simulink model "autopilota_v_15_last"  (R2020b)
settings: Solver=ode4  StartTime=0.0  StopTime=300  FixedStep=0.02  RelTol=1e-3
values from neighbouring files (symbols this model uses):
  attuatore_Amax = 20*(pi/180)    (= 0.349065850399)    [v2021_10_27_avvioSITL.m]    (also in v2021_10_27_calcoloAerodinamica.m)
  attuatore_Amin = -20*(pi/180)    (= -0.349065850399)    [v2021_10_27_avvioSITL.m]
  attuatore_Emax = 25*(pi/180)    (= 0.436332312999)    [v2021_10_27_avvioSITL.m]    (also in v2021_10_27_calcoloAerodinamica.m)
  attuatore_Emin = -25*(pi/180)    (= -0.436332312999)    [v2021_10_27_avvioSITL.m]
  attuatore_Rmax = 25*(pi/180)    (= 0.436332312999)    [v2021_10_27_avvioSITL.m]    (also in v2021_10_27_calcoloAerodinamica.m)
  attuatore_Rmin = -25*(pi/180)    (= -0.436332312999)    [v2021_10_27_avvioSITL.m]
  attuatore_Tmax = 0.99    [v2021_10_27_avvioSITL.m]
  attuatore_Tmin = 0    [v2021_10_27_avvioSITL.m]
  bias = [baccxINI,baccyINI,bacczINI,bpINI,bqINI,brINI]    [v2021_10_27_avvioSITL.m]
  final_h = 35    [v2021_10_27_avvioSITL.m]
  interventoA_05 = 20*0.8    (= 16)    [v2021_10_27_avvioSITL.m]
  interventoA_1 = 10    [v2021_10_27_avvioSITL.m]
  interventoE_05 = 25*0.8    (= 20)    [v2021_10_27_avvioSITL.m]
  interventoE_1 = 10    [v2021_10_27_avvioSITL.m]
  interventoT = 1*0.6    (= 0.6)    [v2021_10_27_avvioSITL.m]
  inv_A = 1    [v2021_10_27_avvioSITL.m]
  inv_comp_h = 1    [v2021_10_27_avvioSITL.m]
  inv_E = 1    [v2021_10_27_avvioSITL.m]
  inv_R = 1    [v2021_10_27_avvioSITL.m]
  inv_T = 1    [v2021_10_27_avvioSITL.m]
  K_AW_B_AP_quota = 1000    [v2021_10_27_avvioSITL.m]
  K_AW_B_becc = -250    [v2021_10_27_avvioSITL.m]
  K_AW_B_imb = 0    [v2021_10_27_avvioSITL.m]
  K_AW_B_roll = 500    [v2021_10_27_avvioSITL.m]
  K_imb_inv = -0.001306    [v2021_10_27_avvioSITL.m]
  Kd_AP_rotta = 0.995    [v2021_10_27_avvioSITL.m]
  Kd_h_app = 0.085    [v2021_10_27_avvioSITL.m]
  Kd_h_flare = 0.01    [v2021_10_27_avvioSITL.m]
  Ki_AP_quota_select = 0.01936    [v2021_10_27_avvioSITL.m]
  Ki_AP_rotta = 0.002    [v2021_10_27_avvioSITL.m]
  Ki_AP_vel = 0.025175    [v2021_10_27_avvioSITL.m]
  Ki_becch = -0.1963    [v2021_10_27_avvioSITL.m]
  Ki_h_app = 0.055    [v2021_10_27_avvioSITL.m]
  Ki_h_cruise = 0.008    [v2021_10_27_avvioSITL.m]
  Ki_h_flare = 0.07    [v2021_10_27_avvioSITL.m]
  Ki_roll = 0.004528    [v2021_10_27_avvioSITL.m]
  Kp_AP_quota_hold_h = 0.5503    [v2021_10_27_avvioSITL.m]
  Kp_AP_quota_hold_l = 0.5503    [v2021_10_27_avvioSITL.m]
  Kp_AP_quota_select = 0.02647    [v2021_10_27_avvioSITL.m]
  Kp_AP_rotta = 0.520    (= 0.52)    [v2021_10_27_avvioSITL.m]
  Kp_AP_vel = 0.132175    [v2021_10_27_avvioSITL.m]
  Kp_becch = -0.30    (= -0.3)    [v2021_10_27_avvioSITL.m]
  Kp_comp_h = 0.035    [v2021_10_27_avvioSITL.m]
  Kp_h_app_max = 0.086    [v2021_10_27_avvioSITL.m]
  Kp_h_app_min = 0.01    [v2021_10_27_avvioSITL.m]
  Kp_h_cruise = 0.04    [v2021_10_27_avvioSITL.m]
  Kp_h_flare = 0.1    [v2021_10_27_avvioSITL.m]
  Kp_imb = 0.0019415    [v2021_10_27_avvioSITL.m]
  Kp_p = 0.006913    [v2021_10_27_avvioSITL.m]
  Kp_q = -0.025    [v2021_10_27_avvioSITL.m]
  Kp_roll = 0.0718    [v2021_10_27_avvioSITL.m]
  Kp_Rotta_ATO = 4    [v2021_10_27_avvioSITL.m]
  Kp_Rotta_psi = -0.01    [v2021_10_27_avvioSITL.m]
  Q1B = [    2e-15;     2e-15 ... (first row only)    [COV_F1B.m]
  R1B = [     2e-14;             2e-14 ... (first row only)    [COV_F1B.m]
  safe_phi = 55    [v2021_10_27_avvioSITL.m]
  safe_V = 40    [v2021_10_27_avvioSITL.m]
  Sensor_Offsets = [0,0,0]    [v2021_10_27_avvioSITL.m]
  T_cal = 0.4    [v2021_10_27_avvioSITL.m]
  theta_rot = 10    [v2021_10_27_avvioSITL.m]
  time_alarm_SAFE = 300    [v2021_10_27_avvioSITL.m]
  tsamp = 0.02    [v2021_10_27_avvioSITL.m]
  update = [2,2,2]    [v2021_10_27_avvioSITL.m]
  V_max = 35    [v2021_10_27_avvioSITL.m]
  V_stall = 15    [v2021_10_27_avvioSITL.m]
  vd_ini = 0    [v2021_10_27_avvioSITL.m]
  vel_wp1_al = 25    [v2021_10_27_avvioSITL.m]
  vel_wp2_al = 20    [v2021_10_27_avvioSITL.m]
undefined symbols (not defined in the file or in its folder): DiscIntNeverNeededParam, Newton, Raphson, t_AP
libraries: simulink_extras x41, pid_lib x8, dspsigops x4, simulink x3, aerolibtransform2sys x2, aerolibtransform2 x2, cstblocks x1, aerosimlib x1
(part 9 of 11)

== matlab function autopilota_v_15_last/Subsystem1/Subsystem1/Subsystem2/WAYPOINTS3 ==
  data: lat input; long input; h input; psi input; WP_db_info input; e_h output; vel output; lat_comandato output; long_comandato output; distance output; QUOTA output; ROTTA output; WP_db_param input; GC_info input; counter input; counter_out output
% % % % function [e_h,vel,lat_comandato,long_comandato,distance,QUOTA,ROTTA,...
% % % %     counter_out] = waypoints_tracking(lat,long,h,psi,WP_db_info,...
% % % %     WP_db_param,GC_info,counter)
% % % % %#codegen
% % % % %WP_db_info=(nWP_tot , n_WP , frame , command , current , autocontinue)
% % % % %per Nav
% % % % %WP_db_param=(velocità, autocontinue, vuoto, vuoto, lat_comandato, ...
% % % % %long_comandato, h_comandato)
% % % % % 
% % % % persistent flag lat1 long1 
% % % % 
% % % % if isempty (flag)
% % % %     flag = 0;
% % % % end
% % % % if isempty (lat1)
% % % %     lat1 = 0;
% % % % end
% % % % if isempty (long1)
% % % %     long1=0;
% % % % end
% % % % 
% % % % % autocontinue = WP_db_param(counter,4);      
% % % % %se vale 1 si procede al waypoint successivo, 
% % % % %se vale 0 loitera sul waypoint
% % % % 
% % % % autocontinue = 1;
% % % % %se arrivo all'ultimo WP, loiter 
% % % % if counter == size(WP_db_param,1) && autocontinue > 0    
% % % %     autocontinue = 0;     
% % % % end
% % % % % if autocontinue >=1
% % % % %     autocontinue = 1;
% % % % % end
% % % % 
% % % % %se ricevo dei WP, comincio dal WP con il current
% % % % %altrimenti ricomincio dal WP1!!!
% % % % if GC_info==3
% % % %     counter=1;
% % % %     lat1=lat;
% % % %     long1=long;
% % % %     for indice=1:size(WP_db_param,1)
% % % %         if WP_db_info(indice,5)==1
% % % %             counter=indice;
% % % %         end
% % % %     end
% % % % end
% % % % 
% % % % %Definizione posizione waypoints
% % % % lat_comandato = WP_db_param(counter,5);
% % % % long_comandato = WP_db_param(counter,6);
% % % % h_comandato = WP_db_param(counter,7);
% % % % Rearth=6378137; %m
% % % % % e_lat = lat_comandato - lat;        %errore in gradi
% % % % % e_long = long_comandato - long;     %errore in gradi 
% % % % e_h = h_comandato - h;
% % % % 
% % % % a = (sin(((lat_comandato-lat)*pi/180)/2))^2+cos(lat*pi/180)*...
% % % %     cos(lat_comandato*pi/180)*(sin(((long_comandato-long)*pi/180)/2))^2;
% % % % c = 2*atan2(sqrt(a),sqrt(1-a));
% % % % distance = Rearth*c;               %distanza velivolo-WP
% % % % 
% % % % if counter > 1
% % % %     psi_ref = atan2(sin((WP_db_param(counter,6)-...
% % % %         WP_db_param(counter-1,6))*pi/180)*...
% % % %         cos(WP_db_param(counter,5)*pi/180),cos(WP_db_param(counter-1,5)...
% % % %         *pi/180)*sin(WP_db_param(counter,5)*pi/180)-...
% % % %         sin(WP_db_param(counter-1,5)*pi/180)*cos(WP_db_param(counter,5)...
% % % %         *pi/180)*cos((WP_db_param(counter,6)-WP_db_param(counter-1,6))...
% % % %         *pi/180))*180/pi;     %psi di riferimento
% % % % %    distWP = sqrt((6378137*(lat_comandato-WP_db_param(counter-1,5))...
% % % % %    *pi/180)^2 + (6378137*(long_comandato-WP_db_param(counter-1,6))...
% % % % %    *pi/180)^2);                          %distanza tra due WP successivi
% % % %     a_pre = (sin(((lat-WP_db_param(counter-1,5))*pi/180)/2))^2+...
% % % %         cos(WP_db_param(counter-1,5)*pi/180)*cos(lat*pi/180)*...
% % % %         (sin(((long-WP_db_param(counter-1,6))*pi/180)/2))^2;
% % % %     c_pre = 2*atan2(sqrt(a_pre),sqrt(1-a_pre));
% % % %     dist = Rearth*c_pre;                  %distanza velivolo-WP precedente
% % % % else
% % % %     psi_ref = atan2(sin((long_comandato-long1)*pi/180)*...
% % % %         cos(lat_comandato*pi/180),cos(lat1*pi/180)*...
% % % %         sin(lat_comandato*pi/180)-sin(lat1*pi/180)*...
% % % %         cos(lat_comandato*pi/180)*cos((long_comandato-long1)...
% % % %         *pi/180))*180/pi;
% % % % %    distWP = 6378137;
% % % %     dist = 0;
% % % % end
% % % % 
% % % % if psi_ref < 0
% % % %     psi_ref = 360 - abs(psi_ref);
% % % % end
% % % %       
% % % % 
% % % % %Definizione angolo tra WP successivi
% % % % if autocontinue == 1
% % % %     a_fut = (sin(((WP_db_param(counter+1,5)-WP_db_param(counter,5))...
% % % %         *pi/180)/2))^2+cos(WP_db_param(counter,5)*pi/180)...
% % % %         *cos(WP_db_param(counter+1,5)*pi/180)...
% % % %         *(sin(((WP_db_param(counter+1,6)-WP_db_param(counter,6))...
% % % %         *pi/180)/2))^2;
% % % %     c_fut = 2*atan2(sqrt(a_fut),sqrt(1-a_fut));
% % % %     dist_fut = 6378137*c_fut;
% % % %     psi_ref_fut = atan2(sin((WP_db_param(counter+1,6)-...
% % % %         WP_db_param(counter,6))*pi/180)*cos(WP_db_param(counter+1,5)...
% % % %         *pi/180),cos(WP_db_param(counter,5)*pi/180)*...
% % % %         sin(WP_db_param(counter+1,5)*pi/180)-sin(WP_db_param(counter,5)...
% % % %         *pi/180)*cos(WP_db_param(counter+1,5)*pi/180)*...
% % % %         cos((WP_db_param(counter+1,6)-WP_db_param(counter,6))...
% % % %         *pi/180))*180/pi;      %distanza WP-WP+1
% % % %     if psi_ref_fut < 0
% % % %         psi_ref_fut = 360 - abs(psi_ref_fut);
% % % %     end
% % % %     if counter > 1
% % % %         angoloWP = abs(psi_ref_fut - psi_ref);
% % % %     else 
% % % %         angoloWP = abs(psi_ref_fut - (atan2(sin((long_comandato-long1)...
% % % %             *pi/180)*cos(lat_comandato*pi/180),cos(lat1*pi/180)*...
% % % %             sin(lat_comandato*pi/180)-sin(lat1*pi/180)*...
% % % %             cos(lat_comandato*pi/180)*cos((long_comandato-long1)...
% % % %             *pi/180))*180/pi));
% % % %     end
% % % % else
% % % %     dist_fut = 0;
% % % %     angoloWP = 0;
% % % % end
% % % % 
% % % % 
% % % % 
% % % % if counter < 2
% % % %     angoloWP_pre = 0;
% % % % elseif counter == 2
% % % %     angoloWP_pre = abs(psi_ref - atan2(sin((WP_db_param(counter-1,6)...
% % % %         -long1)*pi/180)*cos(WP_db_param(counter-1,5)*pi/180),...
% % % %         cos(lat1*pi/180)*sin(WP_db_param(counter-1,5)*pi/180)...
% % % %         -sin(lat1*pi/180)*cos(WP_db_param(counter-1,5)*pi/180)...
% % % %         *cos((WP_db_param(counter-1,6)-long1)*pi/180))*180/pi);
% % % % else
% % % %     psi_ref_pre = atan2(sin((WP_db_param(counter-1,6)-...
% % % %         WP_db_param(counter-2,6))*pi/180)*cos(WP_db_param(counter-1,5)...
% % % %         *pi/180),cos(WP_db_param(counter-2,5)*pi/180)*...
% % % %         sin(WP_db_param(counter-1,5)*pi/180)-...
% % % %         sin(WP_db_param(counter-2,5)*pi/180)*...
% % % %         cos(WP_db_param(counter-1,5)*pi/180)*...
% % % %         cos((WP_db_param(counter-1,6)-WP_db_param(counter-2,6))...
% % % %         *pi/180))*180/pi;
% % % % if psi_ref_pre < 0
% % % %     psi_ref_pre = 360 - abs(psi_ref_pre);
% % % % end
% % % %     angoloWP_pre = abs(psi_ref - psi_ref_pre);
% % % % end
% % % %     
% % % % 
% % % % if angoloWP <= 10
% % % %     error = 40;                            %Definizione raggio di errore 
% % % %     tolleranza_distWP_fut = 100;           %Definizione distanza minima... 
% % % % elseif angoloWP > 10 && angoloWP <= 50     %accettabile tra WP successivi
% % % %     error = 60;
% % % %     tolleranza_distWP_fut = 250;
% % % % elseif angoloWP > 50 && angoloWP <= 90     
% % % %     error = 80;
% % % %     tolleranza_distWP_fut = 300;
% % % % elseif angoloWP > 90 && angoloWP <= 120     
% % % %     error = 120;
% % % %     tolleranza_distWP_fut = 350;
% % % % else     
% % % %     error = 150;
% % % %     tolleranza_distWP_fut = 400;
% % % % end
% % % % 
% % % % %Protezione WP troppo vicini
% % % % % for i=1 : size(WP_db_param,1)-1
% % % % %     a_fut(i) = (sin(((WP_db_param(i+1,5)-WP_db_param(i,5))*pi/180)/2))^2+cos(WP_db_param(i,5)*pi/180)*cos(WP_db_param(i+1,5)*pi/180)*(sin(((WP_db_param(i+1,6)-WP_db_param(i,6))*pi/180)/2))^2;
% % % % %     c_fut(i) = 2*atan2(sqrt(a_fut(i)),sqrt(1-a_fut(i)));
% % % % %     dist_fut(i) = 6378137*c_fut(i);
% % % % %     if dist_fut(i) <= tolleranza_distWP_fut
% % % % %         WP_db_param(i+1,:) = [];
% % % % %     end
% % % % % end
% % % % 
% % % % nWP=size(WP_db_param,1);
% % % % 
% % % % if angoloWP_pre <= 10
% % % % %     tolleranza_distWP = 100;                          
% % % %     soglia_dist = 50;%Distanza dal WP precedente per correzione traiettoria
% % % % elseif angoloWP_pre > 10 && angoloWP_pre <= 50 
% % % % %     tolleranza_distWP = 250;
% % % %     soglia_dist = 200;
% % % % elseif angoloWP_pre > 50 && angoloWP_pre <= 90 
% % % % %     tolleranza_distWP = 300;
% % % %     soglia_dist = 300;
% % % % elseif angoloWP_pre > 90 && angoloWP_pre <= 120 
% % % % %     tolleranza_distWP = 350;
% % % %     soglia_dist = 350;
% % % % else
% % % % %     tolleranza_distWP = 400;
% % % %     soglia_dist = 400;
% % % % end
% % % % 
% % % % k=1.3;    %fattore moltiplicativo correzione rotta
% % % % 
% % % % %Definizione rotta
% % % % 
% % % % if autocontinue == 1
% % % %     
% % % %     psi_comandato = atan2(sin((long_comandato - long)*pi/180)*...
% % % %         cos(lat_comandato*pi/180),cos(lat*pi/180)*...
% % % %         sin(lat_comandato*pi/180)-sin(lat*pi/180)*...
% % % %         cos(lat_comandato*pi/180)*cos((long_comandato - long)...
% % % %         *pi/180))*180/pi;     %rotta da seguire
% % % %     vel = WP_db_param(counter,3);    %??     %inserisci velocità desiderata 
% % % %     psi_comandato_fut = atan2(sin((WP_db_param(counter+1,6)-long)...
% % % %         *pi/180)*cos(WP_db_param(counter+1,5)*pi/180),cos(lat*pi/180)...
% % % %         *sin(WP_db_param(counter+1,5)*pi/180)-sin(lat*pi/180)...
% % % %         *cos(WP_db_param(counter+1,5)*pi/180)...
% % % %         *cos((WP_db_param(counter+1,6)-long)*pi/180))*180/pi;
% % % %     if vel < 15
% % % %         vel = 25;
% % % %     end
% % % %     
% % % %     if vel <= 20%Definizione raggio di errore in base alla velocità di volo
% % % %         error = error*1;
% % % %     elseif (vel <= 25 && vel > 20)
% % % %         error = error*1.2;
% % % %     elseif (vel <= 30 && vel > 25)
% % % %         error = error*1.3;
% % % %     else 
% % % %         error = error*1.4;
% % % %     end
% % % %     
% % % % %         psi_comandato = atan2(sin((long_comandato - long)*pi/180)...
% % % % %             *cos(lat_comandato*pi/180),cos(lat*pi/180)...
% % % % %             *sin(lat_comandato*pi/180)-sin(lat*pi/180)...
% % % % %             *cos(lat_comandato*pi/180)*cos((long_comandato - long)...
% % % % %             *pi/180))*180/pi;    %già dichiarata
% % % % %         if dist < soglia_dist && distance > error
% % % % %             psi_comandato = atan2(sin((long_comandato - long)*pi/180)...
% % % % %                 *cos(lat_comandato*pi/180),cos(lat*pi/180)...
% % % % %                 *sin(lat_comandato*pi/180)-sin(lat*pi/180)...
% % % % %                 *cos(lat_comandato*pi/180)*cos((long_comandato - long)...
% % % % %                 *pi/180))*180/pi;
% % % %          if dist > soglia_dist && distance > error
% % % %             psi_comandato = atan2(sin((long_comandato - long)*pi/180)...
% % % %                 *cos(lat_comandato*pi/180),cos(lat*pi/180)...
% % % %                 *sin(lat_comandato*pi/180)-sin(lat*pi/180)...
% % % %                 *cos(lat_comandato*pi/180)*cos((long_comandato - long)...
% % % %                 *pi/180))*180/pi;
% % % %             err = abs ( psi_comandato - psi_ref );%errore inseguimento rotta
% % % %             if (psi_ref <= 90 && psi_ref >= 0)    %primo quadrante
% % % %                 if psi_comandato > psi_ref
% % % %                     psi_comandato = psi_comandato + k*err;
% % % %                 elseif psi_comandato < psi_ref
% % % %                     psi_comandato = psi_comandato - k*err;
% % % %                 else
% % % %                     psi_comandato = psi_comandato;
% % % %                 end                   
% % % %             elseif (psi_ref <= 180 && psi_ref > 90)   %secondo quadrante
% % % %                 if psi_ref*psi_comandato > 0
% % % %                     if psi_comandato > psi_ref || ( psi_comandato < -90 ...
% % % %                             && psi_comandato > -180)
% % % %                         psi_comandato = psi_comandato + k*err;
% % % %                     elseif psi_comandato < psi_ref
% % % %                         psi_comandato = psi_comandato - k*err;
% % % %                     else
% % % %                         psi_comandato = psi_comandato;
% % % %                     end                      
% % % %                 else
% % % %                     err = abs ( 360 - abs(psi_comandato) - psi_ref); 
% % % %                     if psi_comandato > psi_ref || ( psi_comandato < -90 ...
% % % %                             && psi_comandato > -180)
% % % %                         psi_comandato = psi_comandato + k*err;
% % % %                     elseif psi_comandato < psi_ref
% % % %                         psi_comandato = psi_comandato - k*err;
% % % %                     else
% % % %                         psi_comandato = psi_comandato;
% % % %                     end                     
% % % %                 end
% % % %             elseif(psi_ref < -90 && psi_ref >= -180)       %terzo quadrante
% % % %                 if psi_ref*psi_comandato > 0
% % % %                     if psi_comandato > psi_ref
% % % %                         psi_comandato = psi_comandato + k*err;
% % % %                     elseif psi_comandato < psi_ref  || (psi_comandato <...
% % % %                             180 && psi_comandato > 90)
% % % %                         psi_comandato = psi_comandato - k*err;
% % % %                     else
% % % %                         psi_comandato = psi_comandato;
% % % %                     end  
% % % %                 else
% % % %                     err = abs ( 360 -(psi_comandato) - abs(psi_ref)); 
% % % %                     if psi_comandato > psi_ref
% % % %                         psi_comandato = psi_comandato + k*err;
% % % %                     elseif psi_comandato < psi_ref || (psi_comandato <...
% % % %                             180 && psi_comandato > 90)
% % % %                         psi_comandato = psi_comandato - k*err;
% % % %                     else
% % % %                         psi_comandato = psi_comandato;
% % % %                     end                     
% % % %                 end
% % % %             elseif(psi_ref < 0 && psi_ref >= -90)       %quarto quadrante
% % % %                 if psi_comandato > psi_ref
% % % %                     psi_comandato = psi_comandato + k*err;
% % % %                 elseif psi_comandato < psi_ref
% % % %                     psi_comandato = psi_comandato - k*err;
% % % %                 else
% % % %                     psi_comandato = psi_comandato;
% % % %                 end
% % % %             end
% % % %             
% % % %         elseif distance < error
% % % %             if dist_fut > tolleranza_distWP_fut
% % % %                 psi_comandato = psi_comandato_fut;
% % % %                 counter = counter + 1;
% % % %             else
% % % %                 if counter < nWP-1
% % % %                     counter = counter + 2;
% % % %                 else
% % % %                     vel=22;
% % % %                     h_comandato=h+0.4;
% % % %                     psi_comandato=psi+36.6;   
% % % %                     e_h=0;
% % % %                     flag=1;
% % % %                 end
% % % %             end
% % % %         end
% % % %             
% % % %     flag = 0;
% % % %     
% % % % else
% % % %     
% % % %     psi_comandato = atan2(sin((long_comandato - long)*pi/180)...
% % % %         *cos(lat_comandato*pi/180),cos(lat*pi/180)...
% % % %         *sin(lat_comandato*pi/180)-sin(lat*pi/180)...
% % % %         *cos(lat_comandato*pi/180)*cos((long_comandato - long)...
% % % %         *pi/180))*180/pi;
% % % %     vel = WP_db_param(counter,3);        %inserisci velocità desiderata
% % % %     error = 40;
% % % %     if vel < 15
% % % %         vel = 25;
% % % %     end
% % % %     
% % % %         if dist < soglia_dist && flag == 0
% % % %                   psi_comandato = atan2(sin((long_comandato - long)...
% % % %                       *pi/180)*cos(lat_comandato*pi/180),...
% % % %                       cos(lat*pi/180)*sin(lat_comandato*pi/180)...
% % % %                       -sin(lat*pi/180)*cos(lat_comandato*pi/180)...
% % % %                       *cos((long_comandato - long)*pi/180))*180/pi;
% % % %         elseif dist > soglia_dist && distance > error && flag == 0
% % % %                 err = abs ( psi_comandato - psi_ref );        
% % % %                 if (psi_ref <= 90 && psi_ref >= 0)       %primo quadrante
% % % %                     if psi_comandato > psi_ref
% % % %                         psi_comandato = psi_comandato + k*err;
% % % %                     elseif psi_comandato < psi_ref
% % % %                         psi_comandato = psi_comandato - k*err;
% % % %                     else
% % % %                         psi_comandato = psi_comandato;
% % % %                     end 
% % % %                 elseif (psi_ref <= 180 && psi_ref > 90)  %secondo quadrante
% % % %                     if psi_ref*psi_comandato > 0
% % % %                         if psi_comandato > psi_ref || ( psi_comandato <...
% % % %                                 -90 && psi_comandato > -180)
% % % %                             psi_comandato = psi_comandato + k*err;
% % % %                         elseif psi_comandato < psi_ref
% % % %                             psi_comandato = psi_comandato - k*err;
% % % %                         else
% % % %                             psi_comandato = psi_comandato;
% % % %                         end
% % % %                     else
% % % %                         err = abs ( 360 - abs(psi_comandato) - psi_ref); 
% % % %                         if psi_comandato > psi_ref || ( psi_comandato <...
% % % %                                 -90 && psi_comandato > -180)
% % % %                             psi_comandato = psi_comandato + k*err;
% % % %                         elseif psi_comandato < psi_ref
% % % %                             psi_comandato = psi_comandato - k*err;
% % % %                         else
% % % %                             psi_comandato = psi_comandato;
% % % %                         end                     
% % % %                     end
% % % %                 elseif(psi_ref < -90 && psi_ref >= -180)   %terzo quadrante
% % % %                     if psi_ref*psi_comandato > 0
% % % %                         if psi_comandato > psi_ref
% % % %                             psi_comandato = psi_comandato + k*err;
% % % %                         elseif psi_comandato < psi_ref  || ...
% % % %                                 (psi_comandato < 180 && psi_comandato > 90)
% % % %                             psi_comandato = psi_comandato - k*err;
% % % %                         else
% % % %                             psi_comandato = psi_comandato;
% % % %                         end 
% % % %                     else
% % % %                         err = abs ( 360 -(psi_comandato) - abs(psi_ref)); 
% % % %                         if psi_comandato > psi_ref
% % % %                             psi_comandato = psi_comandato + k*err;
% % % %                         elseif psi_comandato < psi_ref || (psi_comandato...
% % % %                                 < 180 && psi_comandato > 90)
% % % %                             psi_comandato = psi_comandato - k*err;
% % % %                         else
% % % %                             psi_comandato = psi_comandato;
% % % %                         end                         
% % % %                     end
% % % %                 elseif(psi_ref < 0 && psi_ref >= -90) %quarto quadrante
% % % %                     if psi_comandato > psi_ref
% % % %                         psi_comandato = psi_comandato + k*err;
% % % %                     elseif psi_comandato < psi_ref
% % % %                         psi_comandato = psi_comandato - k*err;
% % % %                     else
% % % %                         psi_comandato = psi_comandato;
% % % %                     end
% % % %                 end
% % % %                 
% % % %         else            
% % % %                 vel=22;
% % % %                 h_comandato=h+0.4;
% % % %                 psi_comandato=psi+36.6;   
% % % %                 e_h=0;
% % % %                 flag=1;        %con flag=1 l'aereo rimane in loiter...             
% % % %         end                    %senza uscire dal ciclo
% % % %           
% % % % end
% % % % 
% % % % 
% % % % %se ho nWPtotali=0 (lat,long,alt==0), traiettoria circolare
% % % % if lat_comandato == 0 && long_comandato == 0 && h_comandato==0    
% % % %     h_comandato=h+0.3;
% % % %     psi_comandato=psi+36.6;   
% % % %     vel=22;
% % % %     e_h=0;   
% % % % end
% % % % 
% % % % %output  
% % % % QUOTA = h_comandato;
% % % % ROTTA = psi_comandato;
% % % % 
% % % % counter_out=counter;



function [e_h,vel,lat_comandato,long_comandato,distance,QUOTA,ROTTA,counter_out] = waypoints_tracking(lat,long,h,psi,WP_db_info,WP_db_param,GC_info,counter)
%#codegen
%WP_db_info=(nWP_tot n_WP frame command current autocontinue)
%per Nav
%WP_db_param=(velocità, autocontinue, vuoto, vuoto, lat_comandato, long_comandato, h_comandato)

persistent flag lat1 long1 

if isempty (flag)
    flag = 0;
end
if isempty (lat1)
    lat1 = 0;
end
if isempty (long1)
    long1=0;
end

% autocontinue = WP_db_param(counter,4);      %se vale 1 si procede al waypoint successivo, se vale 0 loitera sul waypoint

autocontinue = 1;
%se arrivo all'ultimo WP, loiter 
if counter == size(WP_db_param,1) && autocontinue > 0    
    autocontinue = 0;     
end
% if autocontinue >=1
%     autocontinue = 1;
% end

%se ricevo dei WP, comincio dal WP con il current
%altrimenti ricomincio dal WP1!!!
if GC_info==3
    counter=1;
    lat1=lat;
    long1=long;
    for indice=1:size(WP_db_param,1)
        if WP_db_info(indice,5)==1
            counter=indice;
        end
    end
end

%Definizione posizione waypoints
lat_comandato = WP_db_param(counter,5);
long_comandato = WP_db_param(counter,6);
h_comandato = WP_db_param(counter,7);

% e_lat = lat_comandato - lat;        %errore in gradi
% e_long = long_comandato - long;     %errore in gradi 
e_h = h_comandato - h;

a = (sin(((lat_comandato-lat)*pi/180)/2))^2+cos(lat*pi/180)*cos(lat_comandato*pi/180)*(sin(((long_comandato-long)*pi/180)/2))^2;
c = 2*atan2(sqrt(a),sqrt(1-a));
distance = 6378137*c;               %distanza velivolo-WP

if counter > 1
    psi_ref = atan2(sin((WP_db_param(counter,6)-WP_db_param(counter-1,6))*pi/180)*cos(WP_db_param(counter,5)*pi/180),cos(WP_db_param(counter-1,5)*pi/180)*sin(WP_db_param(counter,5)*pi/180)-sin(WP_db_param(counter-1,5)*pi/180)*cos(WP_db_param(counter,5)*pi/180)*cos((WP_db_param(counter,6)-WP_db_param(counter-1,6))*pi/180))*180/pi;     %psi di riferimento
%    distWP = sqrt((6378137*(lat_comandato-WP_db_param(counter-1,5))*pi/180)^2 + (6378137*(long_comandato-WP_db_param(counter-1,6))*pi/180)^2);                                          %distanza tra due WP successivi
    a_pre = (sin(((lat-WP_db_param(counter-1,5))*pi/180)/2))^2+cos(WP_db_param(counter-1,5)*pi/180)*cos(lat*pi/180)*(sin(((long-WP_db_param(counter-1,6))*pi/180)/2))^2;
    c_pre = 2*atan2(sqrt(a_pre),sqrt(1-a_pre));
    dist = 6378137*c_pre;                                                  %distanza velivolo-WP precedente
else
    psi_ref = atan2(sin((long_comandato-long1)*pi/180)*cos(lat_comandato*pi/180),cos(lat1*pi/180)*sin(lat_comandato*pi/180)-sin(lat1*pi/180)*cos(lat_comandato*pi/180)*cos((long_comandato-long1)*pi/180))*180/pi;
%    distWP = 6378137;
    dist = 0;
end

if psi_ref < 0
    psi_ref = 360 - abs(psi_ref);
end
      

%Definizione angolo tra WP successivi
if autocontinue == 1
    a_fut = (sin(((WP_db_param(counter+1,5)-WP_db_param(counter,5))*pi/180)/2))^2+cos(WP_db_param(counter,5)*pi/180)*cos(WP_db_param(counter+1,5)*pi/180)*(sin(((WP_db_param(counter+1,6)-WP_db_param(counter,6))*pi/180)/2))^2;
    c_fut = 2*atan2(sqrt(a_fut),sqrt(1-a_fut));
    dist_fut = 6378137*c_fut;
    psi_ref_fut = atan2(sin((WP_db_param(counter+1,6)-WP_db_param(counter,6))*pi/180)*cos(WP_db_param(counter+1,5)*pi/180),cos(WP_db_param(counter,5)*pi/180)*sin(WP_db_param(counter+1,5)*pi/180)-sin(WP_db_param(counter,5)*pi/180)*cos(WP_db_param(counter+1,5)*pi/180)*cos((WP_db_param(counter+1,6)-WP_db_param(counter,6))*pi/180))*180/pi;      %distanza WP-WP+1
    if psi_ref_fut < 0
        psi_ref_fut = 360 - abs(psi_ref_fut);
    end
    if counter > 1
        angoloWP = abs(psi_ref_fut - psi_ref);
    else 
        angoloWP = abs(psi_ref_fut - (atan2(sin((long_comandato-long1)*pi/180)*cos(lat_comandato*pi/180),cos(lat1*pi/180)*sin(lat_comandato*pi/180)-sin(lat1*pi/180)*cos(lat_comandato*pi/180)*cos((long_comandato-long1)*pi/180))*180/pi));
    end
else
    dist_fut = 0;
    angoloWP = 0;
end



if counter < 2
    angoloWP_pre = 0;
elseif counter == 2
    angoloWP_pre = abs(psi_ref - atan2(sin((WP_db_param(counter-1,6)-long1)*pi/180)*cos(WP_db_param(counter-1,5)*pi/180),cos(lat1*pi/180)*sin(WP_db_param(counter-1,5)*pi/180)-sin(lat1*pi/180)*cos(WP_db_param(counter-1,5)*pi/180)*cos((WP_db_param(counter-1,6)-long1)*pi/180))*180/pi);
else
    psi_ref_pre = atan2(sin((WP_db_param(counter-1,6)-WP_db_param(counter-2,6))*pi/180)*cos(WP_db_param(counter-1,5)*pi/180),cos(WP_db_param(counter-2,5)*pi/180)*sin(WP_db_param(counter-1,5)*pi/180)-sin(WP_db_param(counter-2,5)*pi/180)*cos(WP_db_param(counter-1,5)*pi/180)*cos((WP_db_param(counter-1,6)-WP_db_param(counter-2,6))*pi/180))*180/pi;
if psi_ref_pre < 0
    psi_ref_pre = 360 - abs(psi_ref_pre);
end
    angoloWP_pre = abs(psi_ref - psi_ref_pre);
end
    

if angoloWP <= 10
    error = 40;                                       %Definizione raggio di errore 
    tolleranza_distWP_fut = 100;                      %Definizione distanza minima accettabile tra WP successivi
elseif angoloWP > 10 && angoloWP <= 50 
    error = 60;
    tolleranza_distWP_fut = 250;
elseif angoloWP > 50 && angoloWP <= 90     
    error = 80;
    tolleranza_distWP_fut = 300;
elseif angoloWP > 90 && angoloWP <= 120     
    error = 120;
    tolleranza_distWP_fut = 350;
else     
    error = 150;
    tolleranza_distWP_fut = 400;
end

%Protezione WP troppo vicini
% for i=1 : size(WP_db_param,1)-1
%     a_fut(i) = (sin(((WP_db_param(i+1,5)-WP_db_param(i,5))*pi/180)/2))^2+cos(WP_db_param(i,5)*pi/180)*cos(WP_db_param(i+1,5)*pi/180)*(sin(((WP_db_param(i+1,6)-WP_db_param(i,6))*pi/180)/2))^2;
%     c_fut(i) = 2*atan2(sqrt(a_fut(i)),sqrt(1-a_fut(i)));
%     dist_fut(i) = 6378137*c_fut(i);
%     if dist_fut(i) <= tolleranza_distWP_fut
%         WP_db_param(i+1,:) = [];
%     end
% end

nWP=size(WP_db_param,1);

if angoloWP_pre <= 10
%     tolleranza_distWP = 100;                          
    soglia_dist = 50;                                   %Distanza dal WP precedente per correzione traiettoria
elseif angoloWP_pre > 10 && angoloWP_pre <= 50 
%     tolleranza_distWP = 250;
    soglia_dist = 200;
elseif angoloWP_pre > 50 && angoloWP_pre <= 90 
%     tolleranza_distWP = 300;
    soglia_dist = 300;
elseif angoloWP_pre > 90 && angoloWP_pre <= 120 
%     tolleranza_distWP = 350;
    soglia_dist = 350;
else
%     tolleranza_distWP = 400;
    soglia_dist = 400;
end

k=1.3;    %fattore moltiplicativo correzione rotta

%Definizione rotta

if autocontinue == 1
    
    psi_comandato = atan2(sin((long_comandato - long)*pi/180)*cos(lat_comandato*pi/180),cos(lat*pi/180)*sin(lat_comandato*pi/180)-sin(lat*pi/180)*cos(lat_comandato*pi/180)*cos((long_comandato - long)*pi/180))*180/pi;     %rotta da seguire
    vel = WP_db_param(counter,3);                   %inserisci velocità desiderata 
    psi_comandato_fut = atan2(sin((WP_db_param(counter+1,6)-long)*pi/180)*cos(WP_db_param(counter+1,5)*pi/180),cos(lat*pi/180)*sin(WP_db_param(counter+1,5)*pi/180)-sin(lat*pi/180)*cos(WP_db_param(counter+1,5)*pi/180)*cos((WP_db_param(counter+1,6)-long)*pi/180))*180/pi;
    if vel < 15
        vel = 25;
    end
    
    if vel <= 20                                    %Definizione raggio di errore in base alla velocità di volo
        error = error*1;
    elseif (vel <= 25 && vel > 20)
        error = error*1.2;
    elseif (vel <= 30 && vel > 25)
        error = error*1.3;
    else 
        error = error*1.4;
    end
    
        psi_comandato = atan2(sin((long_comandato - long)*pi/180)*cos(lat_comandato*pi/180),cos(lat*pi/180)*sin(lat_comandato*pi/180)-sin(lat*pi/180)*cos(lat_comandato*pi/180)*cos((long_comandato - long)*pi/180))*180/pi;    
        if dist < soglia_dist && distance > error
            psi_comandato = atan2(sin((long_comandato - long)*pi/180)*cos(lat_comandato*pi/180),cos(lat*pi/180)*sin(lat_comandato*pi/180)-sin(lat*pi/180)*cos(lat_comandato*pi/180)*cos((long_comandato - long)*pi/180))*180/pi;
        elseif dist > soglia_dist && distance > error
            psi_comandato = atan2(sin((long_comandato - long)*pi/180)*cos(lat_comandato*pi/180),cos(lat*pi/180)*sin(lat_comandato*pi/180)-sin(lat*pi/180)*cos(lat_comandato*pi/180)*cos((long_comandato - long)*pi/180))*180/pi;
            err = abs ( psi_comandato - psi_ref );             %errore inseguimento rotta
            if (psi_ref <= 90 && psi_ref >= 0)                 %primo quadrante
                if psi_comandato > psi_ref
                    psi_comandato = psi_comandato + k*err;
                elseif psi_comandato < psi_ref
                    psi_comandato = psi_comandato - k*err;
                else
                    psi_comandato = psi_comandato;
                end                   
            elseif (psi_ref <= 180 && psi_ref > 90)             %quarto quadrante
                if psi_ref*psi_comandato > 0
                    if psi_comandato > psi_ref || ( psi_comandato < -90 && psi_comandato > -180)
                        psi_comandato = psi_comandato + k*err;
                    elseif psi_comandato < psi_ref
                        psi_comandato = psi_comandato - k*err;
                    else
                        psi_comandato = psi_comandato;
                    end                      
                else
                    err = abs ( 360 - abs(psi_comandato) - psi_ref); 
                    if psi_comandato > psi_ref || ( psi_comandato < -90 && psi_comandato > -180)
                        psi_comandato = psi_comandato + k*err;
                    elseif psi_comandato < psi_ref
                        psi_comandato = psi_comandato - k*err;
                    else
                        psi_comandato = psi_comandato;
                    end                     
                end
            elseif(psi_ref < -90 && psi_ref >= -180)             %terzo quadrante
                if psi_ref*psi_comandato > 0
                    if psi_comandato > psi_ref
                        psi_comandato = psi_comandato + k*err;
                    elseif psi_comandato < psi_ref  || (psi_comandato < 180 && psi_comandato > 90)
                        psi_comandato = psi_comandato - k*err;
                    else
                        psi_comandato = psi_comandato;
                    end  
                else
                    err = abs ( 360 -(psi_comandato) - abs(psi_ref)); 
                    if psi_comandato > psi_ref
                        psi_comandato = psi_comandato + k*err;
                    elseif psi_comandato < psi_ref || (psi_comandato < 180 && psi_comandato > 90)
                        psi_comandato = psi_comandato - k*err;
                    else
                        psi_comandato = psi_comandato;
                    end                     
                end
            elseif(psi_ref < 0 && psi_ref >= -90)             %secondo quadrante
                if psi_comandato > psi_ref
                    psi_comandato = psi_comandato + k*err;
                elseif psi_comandato < psi_ref
                    psi_comandato = psi_comandato - k*err;
                else
                    psi_comandato = psi_comandato;
                end
            end
            
        elseif distance < error
            if dist_fut > tolleranza_distWP_fut
                psi_comandato = psi_comandato_fut;
                counter = counter + 1;
            else
                if counter < nWP-1
                    counter = counter + 2;
                else
                    vel=22;
                    h_comandato=h+0.4;
                    psi_comandato=psi+36.6;   
                    e_h=0;
                    flag=1;
                end
            end
        end
            
    flag = 0;
    
else
    
    psi_comandato = atan2(sin((long_comandato - long)*pi/180)*cos(lat_comandato*pi/180),cos(lat*pi/180)*sin(lat_comandato*pi/180)-sin(lat*pi/180)*cos(lat_comandato*pi/180)*cos((long_comandato - long)*pi/180))*180/pi;
    vel = WP_db_param(counter,3);                   %inserisci velocità desiderata
    error = 40;
    if vel < 15
        vel = 25;
    end
    
        if dist < soglia_dist && flag == 0
                  psi_comandato = atan2(sin((long_comandato - long)*pi/180)*cos(lat_comandato*pi/180),cos(lat*pi/180)*sin(lat_comandato*pi/180)-sin(lat*pi/180)*cos(lat_comandato*pi/180)*cos((long_comandato - long)*pi/180))*180/pi;
        elseif dist > soglia_dist && distance > error && flag == 0
                err = abs ( psi_comandato - psi_ref );        
                if (psi_ref <= 90 && psi_ref >= 0)                 %primo quadrante
                    if psi_comandato > psi_ref
                        psi_comandato = psi_comandato + k*err;
                    elseif psi_comandato < psi_ref
                        psi_comandato = psi_comandato - k*err;
                    else
                        psi_comandato = psi_comandato;
                    end 
                elseif (psi_ref <= 180 && psi_ref > 90)             %quarto quadrante
                    if psi_ref*psi_comandato > 0
                        if psi_comandato > psi_ref || ( psi_comandato < -90 && psi_comandato > -180)
                            psi_comandato = psi_comandato + k*err;
                        elseif psi_comandato < psi_ref
                            psi_comandato = psi_comandato - k*err;
                        else
                            psi_comandato = psi_comandato;
                        end
                    else
                        err = abs ( 360 - abs(psi_comandato) - psi_ref); 
                        if psi_comandato > psi_ref || ( psi_comandato < -90 && psi_comandato > -180)
                            psi_comandato = psi_comandato + k*err;
                        elseif psi_comandato < psi_ref
                            psi_comandato = psi_comandato - k*err;
                        else
                            psi_comandato = psi_comandato;
                        end                     
                    end
                elseif(psi_ref < -90 && psi_ref >= -180)             %terzo quadrante
                    if psi_ref*psi_comandato > 0
                        if psi_comandato > psi_ref
                            psi_comandato = psi_comandato + k*err;
                        elseif psi_comandato < psi_ref  || (psi_comandato < 180 && psi_comandato > 90)
                            psi_comandato = psi_comandato - k*err;
                        else
                            psi_comandato = psi_comandato;
                        end 
                    else
                        err = abs ( 360 -(psi_comandato) - abs(psi_ref)); 
                        if psi_comandato > psi_ref
                            psi_comandato = psi_comandato + k*err;
                        elseif psi_comandato < psi_ref || (psi_comandato < 180 && psi_comandato > 90)
                            psi_comandato = psi_comandato - k*err;
                        else
                            psi_comandato = psi_comandato;
                        end                         
                    end
                elseif(psi_ref < 0 && psi_ref >= -90)             %secondo quadrante
                    if psi_comandato > psi_ref
                        psi_comandato = psi_comandato + k*err;
                    elseif psi_comandato < psi_ref
                        psi_comandato = psi_comandato - k*err;
                    else
                        psi_comandato = psi_comandato;
                    end
                end
                
        else            
                vel=22;
                h_comandato=h+0.4;
                psi_comandato=psi+36.6;   
                e_h=0;
                flag=1;                       %con flag=1 l'aereo rimane in loiter senza uscire dal ciclo            
        end
          
end


%se ho nWPtotali=0 (lat,long,alt==0), traiettoria circolare
if lat_comandato == 0 && long_comandato == 0 && h_comandato==0    
    h_comandato=h+0.3;
    psi_comandato=psi+36.6;   
    vel=22;
    e_h=0;   
end

%output  
QUOTA = h_comandato;
ROTTA = psi_comandato;

counter_out=counter;





% function [e_h,vel,lat_comandato,long_comandato,distance,QUOTA,ROTTA,counter_out] = waypoints_tracking(lat,long,h,psi,WP_db_info,WP_db_param,GC_info,counter)
% %#codegen
% %WP_db_info=(nWP_tot n_WP frame command current autocontinue)
% %per Nav
% %WP_db_param=(velocità, autocontinue, vuoto, vuoto, lat_comandato, long_comandato, h_comandato)
% 
% persistent flag
% 
% if isempty(flag)
%     flag = 0;
% end
% 
% counter_out=counter;
% autocontinue = WP_db_param(counter,2);      %se vale 1 si procede al waypoint successivo, se vale 0 loitera sul waypoint
% 
% if autocontinue >=1
%     autocontinue = 1;
% end
% 
% %se ricevo dei WP, comincio dal WP con il current
% %altrimenti ricomincio dal WP1!!!
% if GC_info==3
%     counter=1;
%     for indice=1:size(WP_db_param,1)
%         if WP_db_info(indice,5)==1
%             counter=indice;
%         end
%     end
% end
% 
% %Definizione posizione waypoints
% lat_comandato = WP_db_param(counter,5);
% long_comandato = WP_db_param(counter,6);
% h_comandato = WP_db_param(counter,7);
% 
% e_lat = lat_comandato - lat;        %errore in gradi
% e_long = long_comandato - long;     %errore in gradi 
% e_h = h_comandato - h;
% 
% e_x=6378137*e_lat*pi/180;           %passo a errore di distanza   %prima si utilizzava per il raggio 6372800;
% e_y=6378137*e_long*pi/180;          %passo a errore di distanza
% distance=sqrt((e_x)^2 + (e_y)^2 + (e_h)^2);
% 
% if counter > 1   
%     psi_ref = atan2((6378137*(WP_db_param(counter,6)-WP_db_param(counter-1,6))*pi/180),(6378137*((WP_db_param(counter,5)-WP_db_param(counter-1,5))*pi/180))) *180/pi;
% else
%     psi_ref = atan2((e_y),(e_x)) *180/pi; 
% end
% 
% if counter > 1
%     dist = sqrt((6378137*(lat_comandato-WP_db_param(counter-1,5)))^2 + (6378137*(long_comandato-WP_db_param(counter-1,6)))^2);
% else
%     dist = 6378137;
% end
%          
% tolleranza_dist = 320;
% tolleranza_rotta_1 = 18;
% tolleranza_rotta_2 = 9;
% tolleranza_rotta_3 = 2;
% 
% %Definizione rotta
% 
% if autocontinue == 1
%     
%     psi_comandato = atan2((e_y),(e_x)) *180/pi; 
%     vel = WP_db_param(counter,1);         %inserisci velocità desiderata
%     
%     if vel <= 20                          %Definizione raggio di errore
%         error = 25;
%     elseif (vel <= 25 && vel > 20)
%         error = 30;
%     elseif (vel <= 30 && vel > 25)
%         error = 40;
%     else 
%         error = 45;
%     end
% 
%     if dist > tolleranza_dist 
%         
%         psi_comandato = atan2((e_y),(e_x)) *180/pi; 
%         
%         if distance >= error*3
%             
%             if (psi_ref <= 90 && psi_ref >= 0)                 %primo quadrante
%                 if abs(psi_comandato - psi_ref) > tolleranza_rotta_1
%                     if psi_comandato > psi_ref
%                         psi_comandato = psi_comandato + 35;
%                     else
%                         psi_comandato = psi_comandato - 35;
%                     end
%                 elseif abs(psi_comandato - psi_ref) > tolleranza_rotta_2 && abs(psi_comandato - psi_ref) < tolleranza_rotta_1
%                     if psi_comandato > psi_ref
%                         psi_comandato = psi_comandato + 12;
%                     else
%                         psi_comandato = psi_comandato - 12;
%                     end
%                 elseif abs(psi_comandato - psi_ref) > tolleranza_rotta_3 && abs(psi_comandato - psi_ref) < tolleranza_rotta_2
%                     if psi_comandato > psi_ref
%                         psi_comandato = psi_comandato + 4;
%                     else
%                         psi_comandato = psi_comandato - 4;
%                     end
%                 end
%             elseif (psi_ref <= 180 && psi_ref > 90)             %secondo quadrante
%                 if psi_ref*psi_comandato > 0
%                     if abs(psi_comandato - psi_ref) > tolleranza_rotta_1
%                         if (psi_comandato > psi_ref) || ( psi_comandato < -90 && psi_comandato > -180)
%                             psi_comandato = psi_comandato + 35;
%                         else
%                             psi_comandato = psi_comandato - 35;
%                         end
%                     elseif abs(psi_comandato - psi_ref) > tolleranza_rotta_2 && abs(psi_comandato - psi_ref) < tolleranza_rotta_1
%                         if psi_comandato > psi_ref || ( psi_comandato < -90 && psi_comandato > -180)
%                             psi_comandato = psi_comandato + 12;
%                         else
%                             psi_comandato = psi_comandato - 12;
%                         end
%                     elseif abs(psi_comandato - psi_ref) > tolleranza_rotta_3 && abs(psi_comandato - psi_ref) < tolleranza_rotta_2
%                         if psi_comandato > psi_ref || ( psi_comandato < -90 && psi_comandato > -180)
%                             psi_comandato = psi_comandato + 4;
%                         else
%                             psi_comandato = psi_comandato - 4;
%                         end
%                     end
%                 else
%                     if abs(360 - abs(psi_comandato) - psi_ref) > tolleranza_rotta_1
%                         if (psi_comandato > psi_ref) || ( psi_comandato < -90 && psi_comandato > -180)
%                             psi_comandato = psi_comandato + 35;
%                         else
%                             psi_comandato = psi_comandato - 35;
%                         end
%                     elseif abs(360 - abs(psi_comandato) - psi_ref) > tolleranza_rotta_2 && abs(psi_comandato - psi_ref) < tolleranza_rotta_1
%                         if psi_comandato > psi_ref || ( psi_comandato < -90 && psi_comandato > -180)
%                             psi_comandato = psi_comandato + 12;
%                         else
%                             psi_comandato = psi_comandato - 12;
%                         end
%                     elseif abs(360 - abs(psi_comandato) - psi_ref) > tolleranza_rotta_3 && abs(psi_comandato - psi_ref) < tolleranza_rotta_2
%                         if psi_comandato > psi_ref || ( psi_comandato < -90 && psi_comandato > -180)
%                             psi_comandato = psi_comandato + 4;
%                         else
%                             psi_comandato = psi_comandato - 4;
%                         end
%                     end
%                 end
%             elseif(psi_ref < -90 && psi_ref >= -180)             %terzo quadrante
%                 if psi_ref*psi_comandato > 0
%                     if abs(psi_comandato - psi_ref) > tolleranza_rotta_1
%                         if psi_comandato > psi_ref
%                             psi_comandato = psi_comandato + 35;
%                         elseif (psi_comandato < psi_ref) || (psi_comandato < 180 && psi_comandato > 90)
%                             psi_comandato = psi_comandato - 35;
%                         end
%                     elseif abs(psi_comandato - psi_ref) > tolleranza_rotta_2 && abs(psi_comandato - psi_ref) < tolleranza_rotta_1
%                         if psi_comandato > psi_ref
%                             psi_comandato = psi_comandato + 12;
%                         elseif (psi_comandato < psi_ref) || (psi_comandato < 180 && psi_comandato > 90)
%                             psi_comandato = psi_comandato - 12;
%                         end
%                     elseif abs(psi_comandato - psi_ref) > tolleranza_rotta_3 && abs(psi_comandato - psi_ref) < tolleranza_rotta_2
%                         if psi_comandato > psi_ref
%                             psi_comandato = psi_comandato + 4;
%                         elseif (psi_comandato < psi_ref) || (psi_comandato < 180 && psi_comandato > 90)
%                             psi_comandato = psi_comandato - 4;
%                         end
%                     end 
%                 else
%                     if abs(360 - psi_comandato - abs(psi_ref)) > tolleranza_rotta_1
%                         if psi_comandato > psi_ref
%                             psi_comandato = psi_comandato + 35;
%                         elseif (psi_comandato < psi_ref) || (psi_comandato < 180 && psi_comandato > 90)
%                             psi_comandato = psi_comandato - 35;
%                         end
%                     elseif abs(360 - psi_comandato - abs(psi_ref)) > tolleranza_rotta_2 && abs(psi_comandato - psi_ref) < tolleranza_rotta_1
%                         if psi_comandato > psi_ref
%                             psi_comandato = psi_comandato + 12;
%                         elseif (psi_comandato < psi_ref) || (psi_comandato < 180 && psi_comandato > 90)
%                             psi_comandato = psi_comandato - 12;
%                         end
%                     elseif abs(360 - psi_comandato - abs(psi_ref)) > tolleranza_rotta_3 && abs(psi_comandato - psi_ref) < tolleranza_rotta_2
%                         if psi_comandato > psi_ref
%                             psi_comandato = psi_comandato + 4;
%                         elseif (psi_comandato < psi_ref) || (psi_comandato < 180 && psi_comandato > 90)
%                             psi_comandato = psi_comandato - 4;
%                         end
%                     end 
%                 end
%             elseif(psi_ref < 0 && psi_ref >= -90)             %quarto quadrante
%                 if abs(psi_comandato - psi_ref) > tolleranza_rotta_1
%                     if psi_comandato > psi_ref
%                         psi_comandato = psi_comandato + 35;
%                     else
%                         psi_comandato = psi_comandato - 35;
%                     end
%                 elseif abs(psi_comandato - psi_ref) > tolleranza_rotta_2 && abs(psi_comandato - psi_ref) < tolleranza_rotta_1
%                     if psi_comandato > psi_ref
%                         psi_comandato = psi_comandato + 12;
%                     else
%                         psi_comandato = psi_comandato - 12;
%                     end
%                 elseif abs(psi_comandato - psi_ref) > tolleranza_rotta_3 && abs(psi_comandato - psi_ref) < tolleranza_rotta_2
%                     if psi_comandato > psi_ref
%                         psi_comandato = psi_comandato + 4;
%                     else
%                         psi_comandato = psi_comandato - 4;
%                     end
%                 end
%             end
%         elseif (distance < error*3 && distance > error)
% 
%             psi_comandato_fut = atan2((6378137*(WP_db_param(counter+1,6)-long)*pi/180),(6378137*((WP_db_param(counter+1,5)-lat)*pi/180))) *180/pi;
% 
%             if (abs(psi_comandato_fut - psi_comandato) > 30 && abs(psi_comandato_fut - psi_comandato) < 60)
% 
%                 vel = 23;
%                 psi_comandato = psi_comandato_fut;
%                 counter = counter + 1;
% 
%             elseif (abs(psi_comandato_fut - psi_comandato) >= 60 && abs(psi_comandato_fut - psi_comandato) < 90) 
% 
%                 vel = 23;
%                 psi_comandato = psi_comandato_fut;
%                 counter = counter + 1;
% 
%             elseif (abs(psi_comandato_fut - psi_comandato) >= 90 && abs(psi_comandato_fut - psi_comandato) < 120)
%                 vel = 23;
%                 psi_comandato = psi_comandato_fut;
%                 counter=counter + 1;
% 
%             elseif abs(psi_comandato_fut - psi_comandato) > 120
% 
%                 vel = 23;
%                 psi_comandato = psi_comandato_fut;
%                 counter=counter + 1;
% 
%             end
%             
%         else
%             counter = counter + 1;
%             
%         end
%         
%     elseif (dist <= tolleranza_dist && dist > 100)
%         if distance >= error
%             
%             psi_comandato = atan2((e_y),(e_x)) *180/pi; 
%             vel = WP_db_param(counter,1);
%         
%         else 
%             
%             counter = counter + 1;
%             
%         end
%         
%     else
%         
%         counter = counter + 1;
%         
%     end
%         
%         
%     flag = 0;
%           
% else
%    
%         
%     
%     error = 35;
%     if dist > tolleranza_dist
%         
%         if (distance > error*2 && flag == 0) 
% 
%             vel = WP_db_param(counter,1);
%             psi_comandato = atan2((e_y),(e_x)) *180/pi;
% 
% 
%             if (psi_ref <= 90 && psi_ref >= 0)                 %primo quadrante
%                 if abs(psi_comandato - psi_ref) > tolleranza_rotta_1
%                     if psi_comandato > psi_ref
%                         psi_comandato = psi_comandato + 35;
%                     else
%                         psi_comandato = psi_comandato - 35;
%                     end
%                 elseif abs(psi_comandato - psi_ref) > tolleranza_rotta_2 && abs(psi_comandato - psi_ref) < tolleranza_rotta_1
%                     if psi_comandato > psi_ref
%                         psi_comandato = psi_comandato + 12;
%                     else
%                         psi_comandato = psi_comandato - 12;
%                     end
%                 elseif abs(psi_comandato - psi_ref) > tolleranza_rotta_3 && abs(psi_comandato - psi_ref) < tolleranza_rotta_2
%                     if psi_comandato > psi_ref
%                         psi_comandato = psi_comandato + 4;
%                     else
%                         psi_comandato = psi_comandato - 4;
%                     end
%                 end
%             elseif (psi_ref <= 180 && psi_ref > 90)             %secondo quadrante
%                 if psi_ref*psi_comandato > 0
%                     if abs(psi_comandato - psi_ref) > tolleranza_rotta_1
%                         if (psi_comandato > psi_ref) || ( psi_comandato < -90 && psi_comandato > -180)
%                             psi_comandato = psi_comandato + 35;
%                         else
%                             psi_comandato = psi_comandato - 35;
%                         end
%                     elseif abs(psi_comandato - psi_ref) > tolleranza_rotta_2 && abs(psi_comandato - psi_ref) < tolleranza_rotta_1
%                         if psi_comandato > psi_ref || ( psi_comandato < -90 && psi_comandato > -180)
%                             psi_comandato = psi_comandato + 12;
%                         else
%                             psi_comandato = psi_comandato - 12;
%                         end
%                     elseif abs(psi_comandato - psi_ref) > tolleranza_rotta_3 && abs(psi_comandato - psi_ref) < tolleranza_rotta_2
%                         if psi_comandato > psi_ref || ( psi_comandato < -90 && psi_comandato > -180)
%                             psi_comandato = psi_comandato + 4;
%                         else
%                             psi_comandato = psi_comandato - 4;
%                         end
%                     end
%                 else
%                     if abs(360 - abs(psi_comandato) - psi_ref) > tolleranza_rotta_1
%                         if (psi_comandato > psi_ref) || ( psi_comandato < -90 && psi_comandato > -180)
%                             psi_comandato = psi_comandato + 35;
%                         else
%                             psi_comandato = psi_comandato - 35;
%                         end
%                     elseif abs(360 - abs(psi_comandato) - psi_ref) > tolleranza_rotta_2 && abs(psi_comandato - psi_ref) < tolleranza_rotta_1
%                         if psi_comandato > psi_ref || ( psi_comandato < -90 && psi_comandato > -180)
%                             psi_comandato = psi_comandato + 12;
%                         else
%                             psi_comandato = psi_comandato - 12;
%                         end
%                     elseif abs(360 - abs(psi_comandato) - psi_ref) > tolleranza_rotta_3 && abs(psi_comandato - psi_ref) < tolleranza_rotta_2
%                         if psi_comandato > psi_ref || ( psi_comandato < -90 && psi_comandato > -180)
%                             psi_comandato = psi_comandato + 4;
%                         else
%                             psi_comandato = psi_comandato - 4;
%                         end
%                     end
%                 end
%             elseif(psi_ref < -90 && psi_ref >= -180)             %terzo quadrante
%                 if psi_ref*psi_comandato > 0
%                     if abs(psi_comandato - psi_ref) > tolleranza_rotta_1
%                         if psi_comandato > psi_ref
%                             psi_comandato = psi_comandato + 35;
%                         elseif (psi_comandato < psi_ref) || (psi_comandato < 180 && psi_comandato > 90)
%                             psi_comandato = psi_comandato - 35;
%                         end
%                     elseif abs(psi_comandato - psi_ref) > tolleranza_rotta_2 && abs(psi_comandato - psi_ref) < tolleranza_rotta_1
%                         if psi_comandato > psi_ref
%                             psi_comandato = psi_comandato + 12;
%                         elseif (psi_comandato < psi_ref) || (psi_comandato < 180 && psi_comandato > 90)
%                             psi_comandato = psi_comandato - 12;
%                         end
%                     elseif abs(psi_comandato - psi_ref) > tolleranza_rotta_3 && abs(psi_comandato - psi_ref) < tolleranza_rotta_2
%                         if psi_comandato > psi_ref
%                             psi_comandato = psi_comandato + 4;
%                         elseif (psi_comandato < psi_ref) || (psi_comandato < 180 && psi_comandato > 90)
%                             psi_comandato = psi_comandato - 4;
%                         end
%                     end 
%                 else
%                     if abs(360 - psi_comandato - abs(psi_ref)) > tolleranza_rotta_1
%                         if psi_comandato > psi_ref
%                             psi_comandato = psi_comandato + 35;
%                         elseif (psi_comandato < psi_ref) || (psi_comandato < 180 && psi_comandato > 90)
%                             psi_comandato = psi_comandato - 35;
%                         end
%                     elseif abs(360 - psi_comandato - abs(psi_ref)) > tolleranza_rotta_2 && abs(psi_comandato - psi_ref) < tolleranza_rotta_1
%                         if psi_comandato > psi_ref
%                             psi_comandato = psi_comandato + 12;
%                         elseif (psi_comandato < psi_ref) || (psi_comandato < 180 && psi_comandato > 90)
%                             psi_comandato = psi_comandato - 12;
%                         end
%                     elseif abs(360 - psi_comandato - abs(psi_ref)) > tolleranza_rotta_3 && abs(psi_comandato - psi_ref) < tolleranza_rotta_2
%                         if psi_comandato > psi_ref
%                             psi_comandato = psi_comandato + 4;
%                         elseif (psi_comandato < psi_ref) || (psi_comandato < 180 && psi_comandato > 90)
%                             psi_comandato = psi_comandato - 4;
%                         end
%                     end 
%                 end
%             elseif(psi_ref < 0 && psi_ref >= -90)             %quarto quadrante
%                 if abs(psi_comandato - psi_ref) > tolleranza_rotta_1
%                     if psi_comandato > psi_ref
%                         psi_comandato = psi_comandato + 35;
%                     else
%                         psi_comandato = psi_comandato - 35;
%                     end
%                 elseif abs(psi_comandato - psi_ref) > tolleranza_rotta_2 && abs(psi_comandato - psi_ref) < tolleranza_rotta_1
%                     if psi_comandato > psi_ref
%                         psi_comandato = psi_comandato + 12;
%                     else
%                         psi_comandato = psi_comandato - 12;
%                     end
%                 elseif abs(psi_comandato - psi_ref) > tolleranza_rotta_3 && abs(psi_comandato - psi_ref) < tolleranza_rotta_2
%                     if psi_comandato > psi_ref
%                         psi_comandato = psi_comandato + 4;
%                     else
%                         psi_comandato = psi_comandato - 4;
%                     end
%                 end
%             end
%             
%         
%         else
% 
%             vel=22;
%             h_comandato=h+0.4;
%             psi_comandato=psi+30;   
%             e_h=0;
%             flag=1;                       %con flag=1 l'aereo rimane in loiter senza uscire dal ciclo
% 
%         end
%        
%     else
%         
%         if (distance > error*2 && flag == 0)
%             
%             psi_comandato = atan2((e_y),(e_x)) *180/pi; 
%             vel = WP_db_param(counter,1);
%             
%         else
%             
%             vel=22;
%             h_comandato=h+0.4;
%             psi_comandato=psi+30;   
%             e_h=0;
%             flag=1;                       %con flag=1 l'aereo rimane in loiter senza uscire dal ciclo
%             
%         end
%         
%     end
%             
% end
% 
% 
% 
% %se ho nWPtotali=0 (lat,long,alt==0), traiettoria circolare
% if lat_comandato == 0 && long_comandato == 0 && h_comandato==0    
%     h_comandato=h+0.4;
%     psi_comandato=psi+20;   
%     vel=22;
%     e_h=0;   
% end
% 
% %output  
% QUOTA = h_comandato;
% ROTTA = psi_comandato;
% 
% 
% %se arrivo all'ultimo WP, loiter 
% if counter == size(WP_db_param,1) && autocontinue > 0    
%     autocontinue = 0;     
% end
% 
% counter_out=counter;
